simulink model "two_tanks_model_cascade_SIMC"  (R2018b)
settings: Solver=FixedStepAuto  StartTime=0.0  StopTime=3600  FixedStep=0.1  RelTol=1e-3
model workspace (MATLAB code in the model file):
  | A1 = 1;
  | a1 = 0.1*0.1;
  | A2 = A1;
  | a2 = a1;
  | h10 = 1;
  | h20=1;
values from neighbouring files (symbols this model uses):
  kc2 = 1    [two_tanks_cascade.m]    (also in two_tanks_cascade_ffwd.m)
  taui2 = t2    (= 59)    [two_tanks_cascade.m]    (also in two_tanks_cascade_ffwd.m)
settings Model: PacingRate=100  Creator=kjartan  LastModifiedBy=kjartan

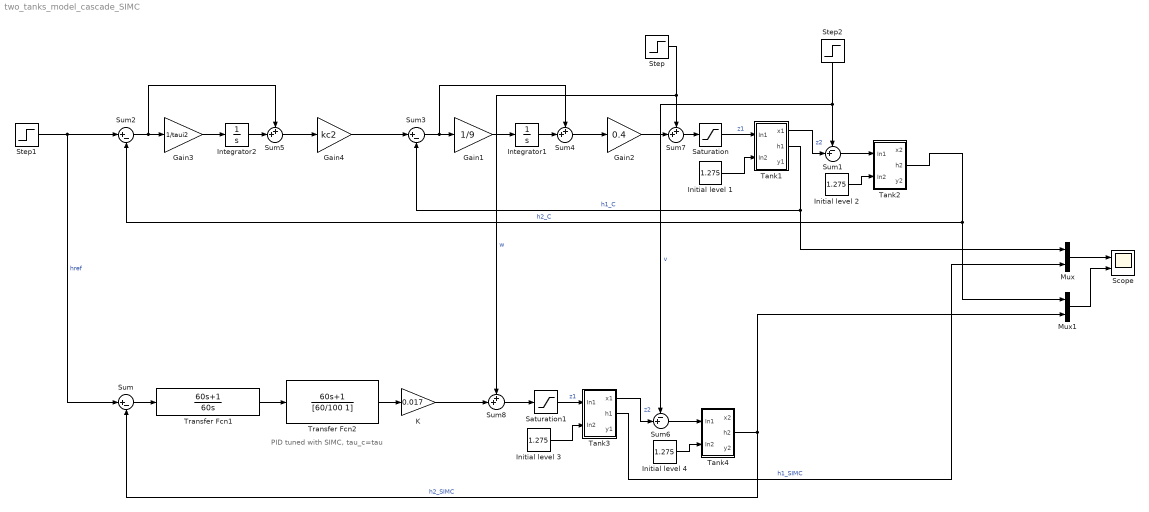
== system two_tanks_model_cascade_SIMC ==
  note: PID tuned with SIMC, tau_c=tau
  Gain1 : Gain  Gain=1/9
  Gain2 : Gain  Gain=0.4
  Gain3 : Gain  Gain=1/taui2
  Gain4 : Gain  Gain=kc2
  Initial level {1..4} (4 alike) : Constant  Value=1.275
  Integrator1 : Integrator
  Integrator2 : Integrator
  K : Gain  Gain=0.017
  Mux : Mux  Inputs=2
  Mux1 : Mux  Inputs=2
  Saturation : Saturate  LowerLimit=0
  Saturation1 : Saturate  LowerLimit=0
  Scope : Scope  NumInputPorts=2
  Step : Step  Time=1600  After=-0.015  SampleTime=0
  Step1 : Step  Time=800  Before=1.275  After=2  SampleTime=0
  Step2 : Step  Time=2400  After=0.015  SampleTime=0
  Sum : Sum  Inputs=|+-
  Sum1 : Sum  Inputs=-+|
  Sum2 : Sum  Inputs=|+-
  Sum3 : Sum  Inputs=|+-
  Sum{4..5,7..8} (4 alike) : Sum  Inputs=++|
  Sum6 : Sum  Inputs=-+|
  Tank1 : Subsystem
  Tank2 : Subsystem
  Tank3 : Subsystem
  Tank4 : Subsystem
  Transfer Fcn1 : TransferFcn  Numerator=[60, 1]  Denominator=[60 0]
  Transfer Fcn2 : TransferFcn  Numerator=[60, 1]  Denominator=[60/100 1]
  wires:
  Tank1/1(x1) -> Sum1/2  "z2"
  Tank1/2(h1) -> Mux/1, Sum3/2  "h1_C"
  Sum1/1 -> Tank2/1(In1)
  Saturation/1 -> Tank1/1(In1)  "z1"
  Initial level 2/1 -> Tank2/2(In2)
  Initial level 1/1 -> Tank1/2(In2)
  Step2/1 -> Sum6/1, Sum1/1  "v"
  Gain1/1 -> Integrator1/1
  Integrator1/1 -> Sum4/2
  Sum3/1 -> Sum4/1, Gain1/1
  Sum4/1 -> Gain2/1
  Gain2/1 -> Sum7/2
  Gain3/1 -> Integrator2/1
  Tank2/2(h2) -> Mux1/1, Sum2/2  "h2_C"
  Gain4/1 -> Sum3/1
  Sum2/1 -> Sum5/1, Gain3/1
  Sum5/1 -> Gain4/1
  Integrator2/1 -> Sum5/2
  Transfer Fcn2/1 -> K/1
  Initial level 3/1 -> Tank3/2(In2)
  Saturation1/1 -> Tank3/1(In1)  "z1"
  Tank3/2(h1) -> Mux/2  "h1_SIMC"
  K/1 -> Sum8/2
  Initial level 4/1 -> Tank4/2(In2)
  Step1/1 -> Sum2/1, Sum/1  "href"
  Sum/1 -> Transfer Fcn1/1
  Sum6/1 -> Tank4/1(In1)
  Tank3/1(x1) -> Sum6/2  "z2"
  Transfer Fcn1/1 -> Transfer Fcn2/1
  Tank4/2(h2) -> Mux1/2, Sum/2  "h2_SIMC"
  Mux/1 -> Scope/1
  Mux1/1 -> Scope/2
  Sum7/1 -> Saturation/1
  Step/1 -> Sum8/1, Sum7/1  "w"
  Sum8/1 -> Saturation1/1

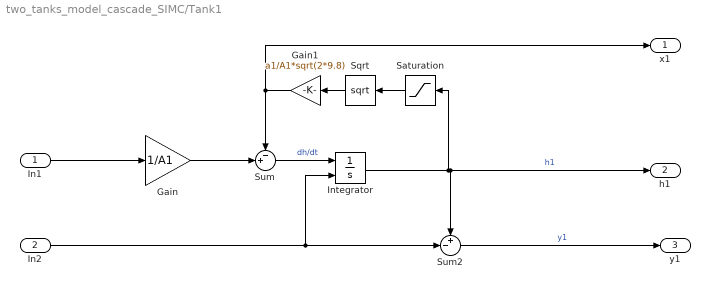
== system two_tanks_model_cascade_SIMC/Tank1 ==
  In1 : Inport
  In2 : Inport  Port=2
  Gain : Gain  Gain=1/A1
  Gain1 : Gain  Gain=a1/A1*sqrt(2*9.8)
  Integrator : Integrator  InitialConditionSource=external  InitialCondition=h10
  Saturation : Saturate  UpperLimit=100  LowerLimit=0
  Sqrt : Sqrt  SaturateOnIntegerOverflow=on
  Sum : Sum  Inputs=-+|
  Sum2 : Sum  Inputs=+-|
  x1 : Outport
  h1 : Outport  Port=2
  y1 : Outport  Port=3
  wires:
  Gain1/1 -> x1/1, Sum/1
  Gain/1 -> Sum/2
  Sum/1 -> Integrator/1  "dh/dt"
  In1/1 -> Gain/1
  Sum2/1 -> y1/1  "y1"
  Sqrt/1 -> Gain1/1
  Integrator/1 -> Saturation/1, h1/1, Sum2/1  "h1"
  In2/1 -> Sum2/2, Integrator/2
  Saturation/1 -> Sqrt/1

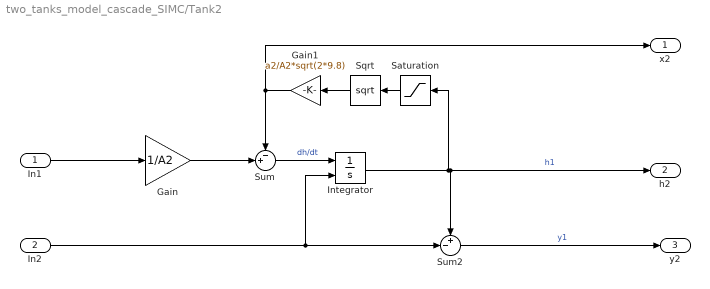
== system two_tanks_model_cascade_SIMC/Tank2 ==
  In1 : Inport
  In2 : Inport  Port=2
  Gain : Gain  Gain=1/A2
  Gain1 : Gain  Gain=a2/A2*sqrt(2*9.8)
  Integrator : Integrator  InitialConditionSource=external  InitialCondition=h10
  Saturation : Saturate  UpperLimit=100  LowerLimit=0
  Sqrt : Sqrt  SaturateOnIntegerOverflow=on
  Sum : Sum  Inputs=-+|
  Sum2 : Sum  Inputs=+-|
  x2 : Outport
  h2 : Outport  Port=2
  y2 : Outport  Port=3
  wires:
  Gain1/1 -> x2/1, Sum/1
  Gain/1 -> Sum/2
  Sum/1 -> Integrator/1  "dh/dt"
  In1/1 -> Gain/1
  Sum2/1 -> y2/1  "y1"
  Sqrt/1 -> Gain1/1
  Integrator/1 -> Saturation/1, h2/1, Sum2/1  "h1"
  In2/1 -> Sum2/2, Integrator/2
  Saturation/1 -> Sqrt/1

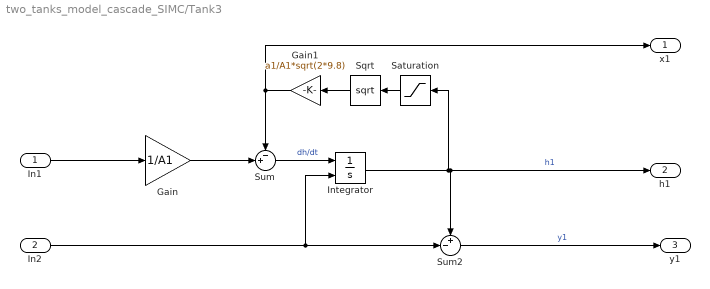
== system two_tanks_model_cascade_SIMC/Tank3 ==
  In1 : Inport
  In2 : Inport  Port=2
  Gain : Gain  Gain=1/A1
  Gain1 : Gain  Gain=a1/A1*sqrt(2*9.8)
  Integrator : Integrator  InitialConditionSource=external  InitialCondition=h10
  Saturation : Saturate  UpperLimit=100  LowerLimit=0
  Sqrt : Sqrt  SaturateOnIntegerOverflow=on
  Sum : Sum  Inputs=-+|
  Sum2 : Sum  Inputs=+-|
  x1 : Outport
  h1 : Outport  Port=2
  y1 : Outport  Port=3
  wires:
  Gain1/1 -> x1/1, Sum/1
  Gain/1 -> Sum/2
  Sum/1 -> Integrator/1  "dh/dt"
  In1/1 -> Gain/1
  Sum2/1 -> y1/1  "y1"
  Sqrt/1 -> Gain1/1
  Integrator/1 -> Saturation/1, h1/1, Sum2/1  "h1"
  Saturation/1 -> Sqrt/1
  In2/1 -> Sum2/2, Integrator/2

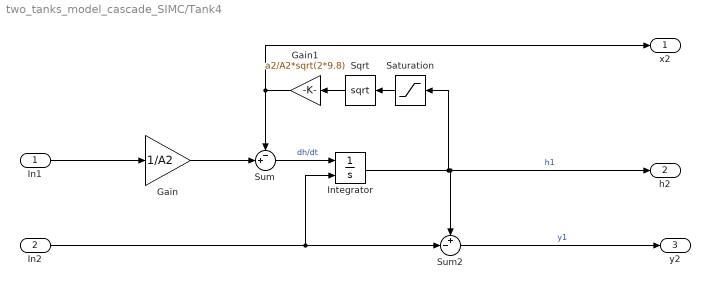
== system two_tanks_model_cascade_SIMC/Tank4 ==
  In1 : Inport
  In2 : Inport  Port=2
  Gain : Gain  Gain=1/A2
  Gain1 : Gain  Gain=a2/A2*sqrt(2*9.8)
  Integrator : Integrator  InitialConditionSource=external  InitialCondition=h10
  Saturation : Saturate  UpperLimit=100  LowerLimit=0
  Sqrt : Sqrt  SaturateOnIntegerOverflow=on
  Sum : Sum  Inputs=-+|
  Sum2 : Sum  Inputs=+-|
  x2 : Outport
  h2 : Outport  Port=2
  y2 : Outport  Port=3
  wires:
  Gain1/1 -> x2/1, Sum/1
  Gain/1 -> Sum/2
  Sum/1 -> Integrator/1  "dh/dt"
  In1/1 -> Gain/1
  Sum2/1 -> y2/1  "y1"
  Integrator/1 -> Saturation/1, h2/1, Sum2/1  "h1"
  In2/1 -> Sum2/2, Integrator/2
  Sqrt/1 -> Gain1/1
  Saturation/1 -> Sqrt/1
